simulink model "systemBrainModel"  (R2024b)
settings: Solver=VariableStepAuto  StartTime=0.0  StopTime=10.0  RelTol=1e-3
settings Model: Creator=roryd  LastModifiedBy=roryd

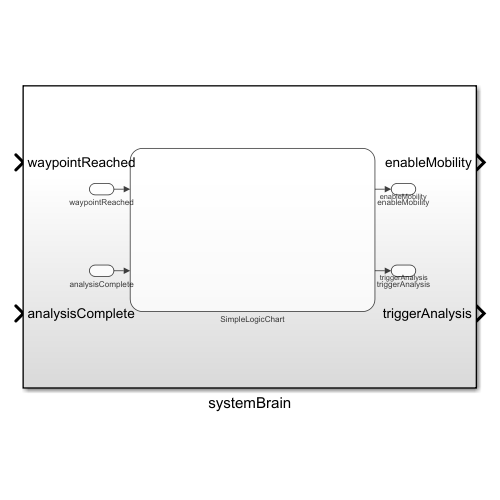
[thumbnail: Simulink's stored preview of the top-level diagram]
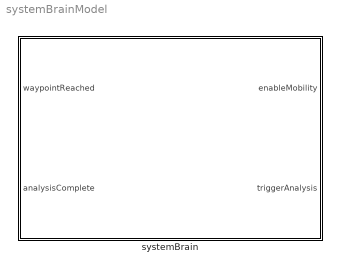
== system systemBrainModel ==
  systemBrain : Subsystem

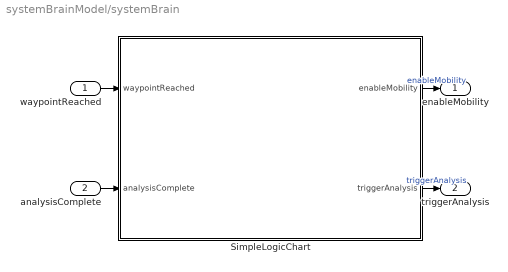
== system systemBrainModel/systemBrain ==
  waypointReached : Inport
  analysisComplete : Inport  Port=2
  SimpleLogicChart : Stateflow chart  TreatAsAtomicUnit=on
  enableMobility : Outport
  triggerAnalysis : Outport  Port=2
  wires:
  waypointReached/1 -> SimpleLogicChart/1(waypointReached)
  analysisComplete/1 -> SimpleLogicChart/2(analysisComplete)
  SimpleLogicChart/1(enableMobility) -> enableMobility/1  "enableMobility"
  SimpleLogicChart/2(triggerAnalysis) -> triggerAnalysis/1  "triggerAnalysis"

== stateflow chart systemBrainModel/systemBrain/SimpleLogicChart ==
  state MoveToWaypoint
    entry: enableMobility = true;
    triggerAnalysis = false;
  state PerformAnalysis
    entry: enableMobility = false;
    triggerAnalysis = true;
  PerformAnalysis -> MoveToWaypoint : [analysisComplete]
  (default) -> MoveToWaypoint
  MoveToWaypoint -> PerformAnalysis : [waypointReached]
  data: waypointReached input boolean; analysisComplete input boolean; enableMobility output boolean; triggerAnalysis output boolean
